simulink model "simulation"  (R2025b)
settings: Solver=VariableStepAuto  StartTime=0.0  StopTime=10.0  RelTol=1e-3
settings Model: Creator=sebas  LastModifiedBy=sebas

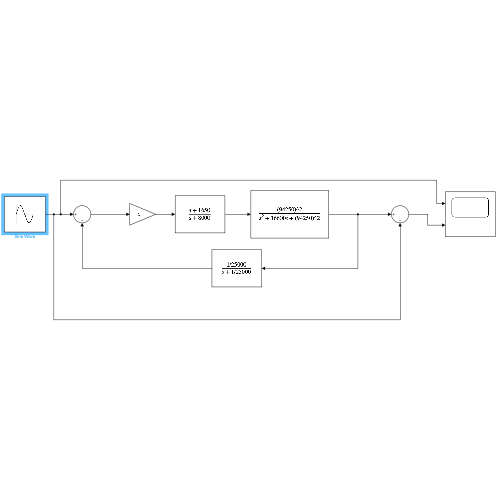
[thumbnail: Simulink's stored preview of the top-level diagram]
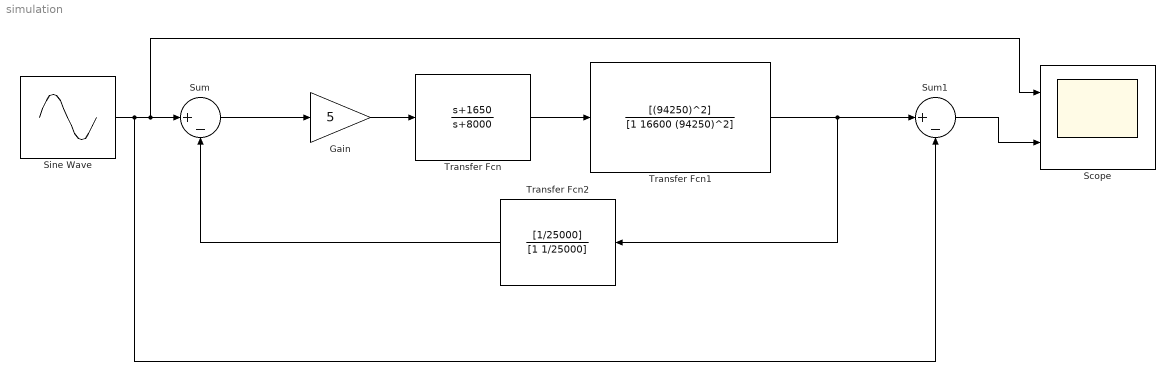
== system simulation ==
  Gain : Gain  Gain=5
  Scope : Scope  NumInputPorts=2
      settings: ActiveDisplayYMinimum=-0.404983522240741  ActiveDisplayYMaximum=1.2087477469353232
  Sine Wave : Sin  Frequency=500  SampleTime=0
  Sum : Sum  Inputs=|+-
  Sum1 : Sum  Inputs=|+-
  Transfer Fcn : TransferFcn  Numerator=[1 1650]  Denominator=[1 8000]
  Transfer Fcn1 : TransferFcn  Numerator=[(94250)^2]  Denominator=[1 16600 (94250)^2]
  Transfer Fcn2 : TransferFcn  Numerator=[1/25000]  Denominator=[1 1/25000]
  wires:
  Transfer Fcn/1 -> Transfer Fcn1/1
  Transfer Fcn1/1 -> Sum1/1, Transfer Fcn2/1
  Transfer Fcn2/1 -> Sum/2
  Sine Wave/1 -> Sum1/2, Scope/1, Sum/1
  Sum1/1 -> Scope/2
  Sum/1 -> Gain/1
  Gain/1 -> Transfer Fcn/1
